simulink model "sensor_diagnosis"  (R2018b)
settings: Solver=FixedStepAuto  StartTime=0.0  StopTime=2000  FixedStep=0.02  RelTol=1e-3
values from neighbouring files (symbols this model uses):
  R = 0.003*eye(size(C,1))    [Com_of_kalman_gain.m]    (also in Copy_of_kalman_gain.m = diag(y_noise.^2); MM_HKF.m = diag(y_svar.^2); MM_based.m = diag(y_svar.^2); act_fault_of_kalman_gain.m = 0.02^2*eye(size(C,1)))
undefined symbols (not defined in the file or in its folder): piece
libraries: sharedschedule x121, dspsigattribs x22, commchan3 x1, dsparch4 x1, simulink x1
(part 2 of 2)

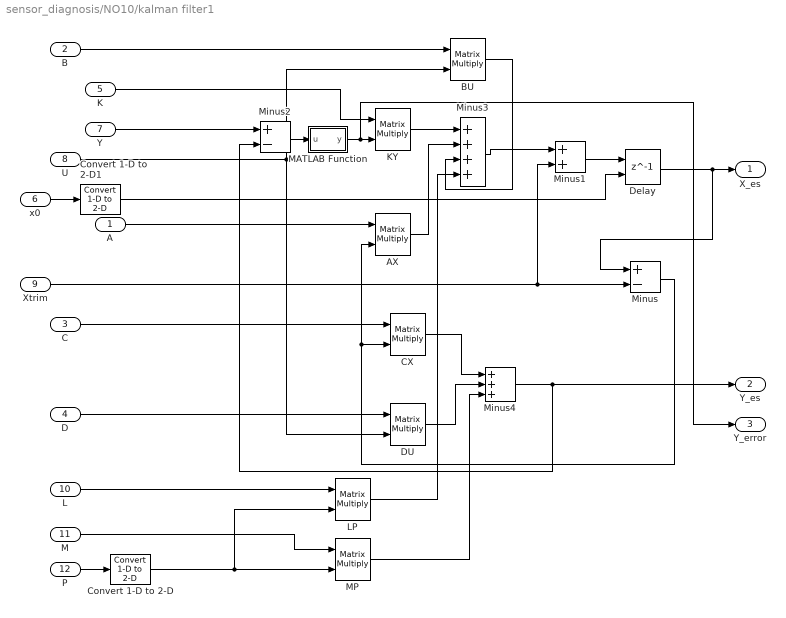
== system sensor_diagnosis/NO10/kalman filter1 ==
  A : Inport
  B : Inport  Port=2
  C : Inport  Port=3
  D : Inport  Port=4
  K : Inport  Port=5
  x0 : Inport  Port=6
  Y : Inport  Port=7
  U : Inport  Port=8
  Xtrim : Inport  Port=9
  L : Inport  Port=10
  M : Inport  Port=11
  P : Inport  Port=12
  "\tCX" : Product  Multiplication=Matrix(*)
  AX : Product  Multiplication=Matrix(*)
  BU : Product  Multiplication=Matrix(*)
  Convert 1-D to 2-D : dspsigattribs/Convert 1-D to 2-D  M=10  N=1  frameBasedOut=off
      settings: SourceProductName=DSP System Toolbox  SourceProductBaseCode=DS
  Convert 1-D to 2-D1 : dspsigattribs/Convert 1-D to 2-D  M=2  N=1  frameBasedOut=off
      settings: SourceProductName=DSP System Toolbox  SourceProductBaseCode=DS
  DU : Product  Multiplication=Matrix(*)
  Delay : Delay  DelayLength=1  InitialConditionSource=Input port
      settings: InputPortMap=u0,p4
  KY : Product  Multiplication=Matrix(*)
  LP : Product  Multiplication=Matrix(*)
  MATLAB Function : MATLAB Function  TreatAsAtomicUnit=on
  MP : Product  Multiplication=Matrix(*)
  Minus : Sum  Inputs=+-
  Minus1 : Sum
  Minus2 : Sum  Inputs=+-
  Minus3 : Sum  Inputs=++++
  Minus4 : Sum  Inputs=+++
  X_es : Outport
  Y_es : Outport  Port=2
  Y_error : Outport  Port=3
  wires:
  Minus1/1 -> Delay/1
  Minus3/1 -> Minus1/1
  AX/1 -> Minus3/2
  Minus/1 -> "\tCX"/2, AX/2
  Delay/1 -> X_es/1, Minus/1
  Xtrim/1 -> Minus/2, Minus1/2
  K/1 -> KY/1
  D/1 -> DU/1
  C/1 -> "\tCX"/1
  B/1 -> BU/1
  A/1 -> AX/1
  BU/1 -> Minus3/3
  "\tCX"/1 -> Minus4/1
  DU/1 -> Minus4/2
  Y/1 -> Minus2/1
  U/1 -> DU/2, BU/2
  KY/1 -> Minus3/1
  Minus4/1 -> Y_es/1, Minus2/2
  L/1 -> LP/1
  M/1 -> MP/1
  LP/1 -> Minus3/4
  MP/1 -> Minus4/3
  P/1 -> Convert 1-D to 2-D/1
  Convert 1-D to 2-D/1 -> LP/2, MP/2
  x0/1 -> Convert 1-D to 2-D1/1
  Convert 1-D to 2-D1/1 -> Delay/2
  Minus2/1 -> MATLAB Function/1(u)
  MATLAB Function/1(y) -> Y_error/1, KY/2

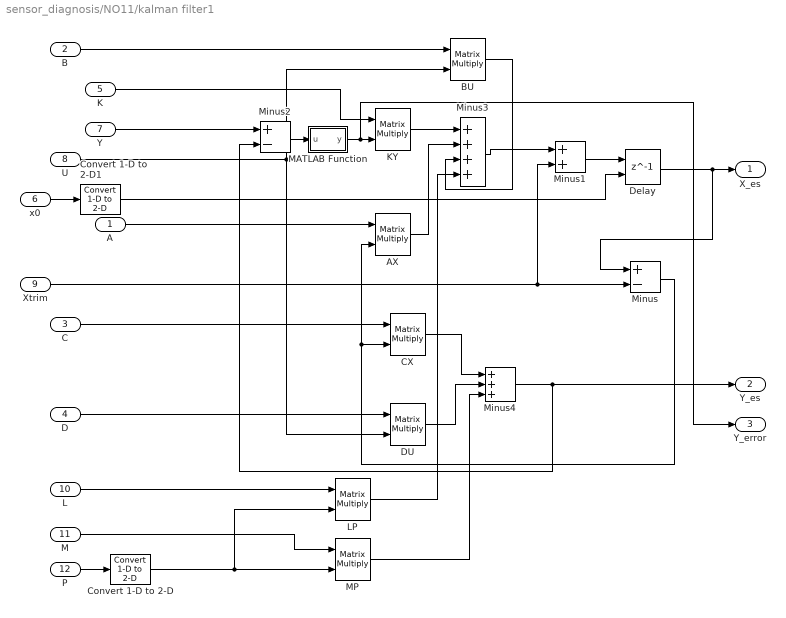
== system sensor_diagnosis/NO11/kalman filter1 ==
  A : Inport
  B : Inport  Port=2
  C : Inport  Port=3
  D : Inport  Port=4
  K : Inport  Port=5
  x0 : Inport  Port=6
  Y : Inport  Port=7
  U : Inport  Port=8
  Xtrim : Inport  Port=9
  L : Inport  Port=10
  M : Inport  Port=11
  P : Inport  Port=12
  "\tCX" : Product  Multiplication=Matrix(*)
  AX : Product  Multiplication=Matrix(*)
  BU : Product  Multiplication=Matrix(*)
  Convert 1-D to 2-D : dspsigattribs/Convert 1-D to 2-D  M=10  N=1  frameBasedOut=off
      settings: SourceProductName=DSP System Toolbox  SourceProductBaseCode=DS
  Convert 1-D to 2-D1 : dspsigattribs/Convert 1-D to 2-D  M=2  N=1  frameBasedOut=off
      settings: SourceProductName=DSP System Toolbox  SourceProductBaseCode=DS
  DU : Product  Multiplication=Matrix(*)
  Delay : Delay  DelayLength=1  InitialConditionSource=Input port
      settings: InputPortMap=u0,p4
  KY : Product  Multiplication=Matrix(*)
  LP : Product  Multiplication=Matrix(*)
  MATLAB Function : MATLAB Function  TreatAsAtomicUnit=on
  MP : Product  Multiplication=Matrix(*)
  Minus : Sum  Inputs=+-
  Minus1 : Sum
  Minus2 : Sum  Inputs=+-
  Minus3 : Sum  Inputs=++++
  Minus4 : Sum  Inputs=+++
  X_es : Outport
  Y_es : Outport  Port=2
  Y_error : Outport  Port=3
  wires:
  MATLAB Function/1(y) -> KY/2, Y_error/1
  Minus2/1 -> MATLAB Function/1(u)
  Convert 1-D to 2-D1/1 -> Delay/2
  x0/1 -> Convert 1-D to 2-D1/1
  Convert 1-D to 2-D/1 -> MP/2, LP/2
  P/1 -> Convert 1-D to 2-D/1
  MP/1 -> Minus4/3
  LP/1 -> Minus3/4
  M/1 -> MP/1
  L/1 -> LP/1
  Minus4/1 -> Minus2/2, Y_es/1
  KY/1 -> Minus3/1
  U/1 -> BU/2, DU/2
  Y/1 -> Minus2/1
  DU/1 -> Minus4/2
  "\tCX"/1 -> Minus4/1
  BU/1 -> Minus3/3
  A/1 -> AX/1
  B/1 -> BU/1
  C/1 -> "\tCX"/1
  D/1 -> DU/1
  K/1 -> KY/1
  Xtrim/1 -> Minus1/2, Minus/2
  Delay/1 -> Minus/1, X_es/1
  Minus/1 -> AX/2, "\tCX"/2
  AX/1 -> Minus3/2
  Minus3/1 -> Minus1/1
  Minus1/1 -> Delay/1

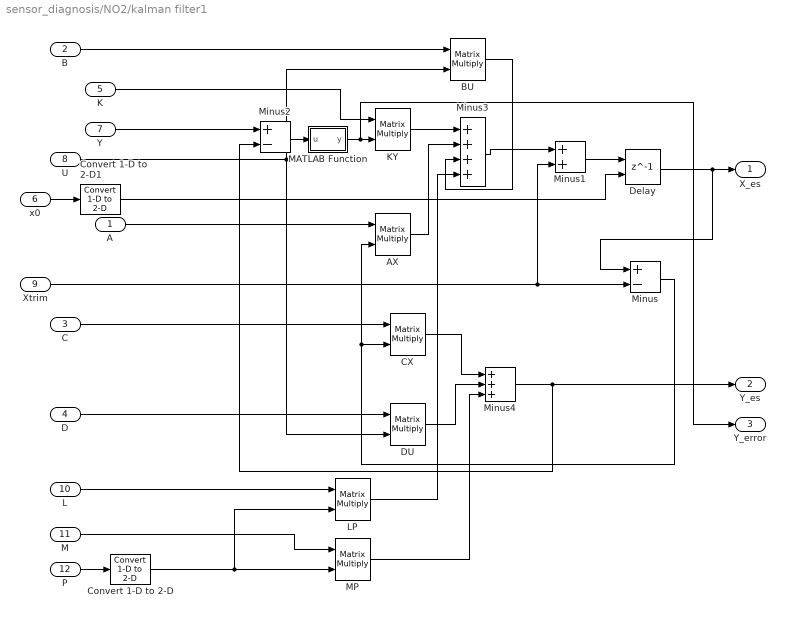
== system sensor_diagnosis/NO2/kalman filter1 ==
  A : Inport
  B : Inport  Port=2
  C : Inport  Port=3
  D : Inport  Port=4
  K : Inport  Port=5
  x0 : Inport  Port=6
  Y : Inport  Port=7
  U : Inport  Port=8
  Xtrim : Inport  Port=9
  L : Inport  Port=10
  M : Inport  Port=11
  P : Inport  Port=12
  "\tCX" : Product  Multiplication=Matrix(*)
  AX : Product  Multiplication=Matrix(*)
  BU : Product  Multiplication=Matrix(*)
  Convert 1-D to 2-D : dspsigattribs/Convert 1-D to 2-D  M=10  N=1  frameBasedOut=off
      settings: SourceProductName=DSP System Toolbox  SourceProductBaseCode=DS
  Convert 1-D to 2-D1 : dspsigattribs/Convert 1-D to 2-D  M=2  N=1  frameBasedOut=off
      settings: SourceProductName=DSP System Toolbox  SourceProductBaseCode=DS
  DU : Product  Multiplication=Matrix(*)
  Delay : Delay  DelayLength=1  InitialConditionSource=Input port
      settings: InputPortMap=u0,p4
  KY : Product  Multiplication=Matrix(*)
  LP : Product  Multiplication=Matrix(*)
  MATLAB Function : MATLAB Function  TreatAsAtomicUnit=on
  MP : Product  Multiplication=Matrix(*)
  Minus : Sum  Inputs=+-
  Minus1 : Sum
  Minus2 : Sum  Inputs=+-
  Minus3 : Sum  Inputs=++++
  Minus4 : Sum  Inputs=+++
  X_es : Outport
  Y_es : Outport  Port=2
  Y_error : Outport  Port=3
  wires:
  Minus1/1 -> Delay/1
  Minus3/1 -> Minus1/1
  AX/1 -> Minus3/2
  Minus/1 -> "\tCX"/2, AX/2
  Delay/1 -> X_es/1, Minus/1
  Xtrim/1 -> Minus/2, Minus1/2
  K/1 -> KY/1
  D/1 -> DU/1
  C/1 -> "\tCX"/1
  B/1 -> BU/1
  A/1 -> AX/1
  BU/1 -> Minus3/3
  "\tCX"/1 -> Minus4/1
  DU/1 -> Minus4/2
  Y/1 -> Minus2/1
  U/1 -> DU/2, BU/2
  KY/1 -> Minus3/1
  Minus4/1 -> Y_es/1, Minus2/2
  L/1 -> LP/1
  M/1 -> MP/1
  LP/1 -> Minus3/4
  MP/1 -> Minus4/3
  P/1 -> Convert 1-D to 2-D/1
  Convert 1-D to 2-D/1 -> LP/2, MP/2
  x0/1 -> Convert 1-D to 2-D1/1
  Convert 1-D to 2-D1/1 -> Delay/2
  Minus2/1 -> MATLAB Function/1(u)
  MATLAB Function/1(y) -> Y_error/1, KY/2

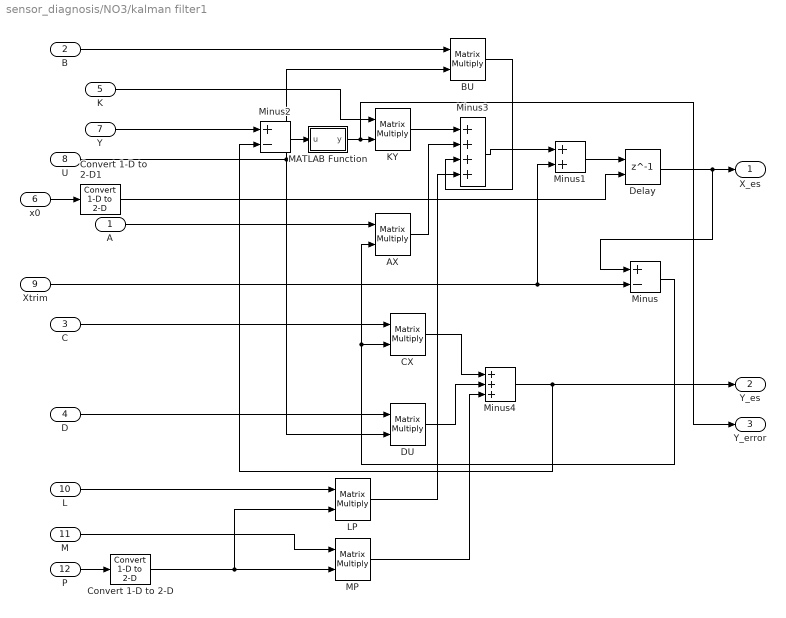
== system sensor_diagnosis/NO3/kalman filter1 ==
  A : Inport
  B : Inport  Port=2
  C : Inport  Port=3
  D : Inport  Port=4
  K : Inport  Port=5
  x0 : Inport  Port=6
  Y : Inport  Port=7
  U : Inport  Port=8
  Xtrim : Inport  Port=9
  L : Inport  Port=10
  M : Inport  Port=11
  P : Inport  Port=12
  "\tCX" : Product  Multiplication=Matrix(*)
  AX : Product  Multiplication=Matrix(*)
  BU : Product  Multiplication=Matrix(*)
  Convert 1-D to 2-D : dspsigattribs/Convert 1-D to 2-D  M=10  N=1  frameBasedOut=off
      settings: SourceProductName=DSP System Toolbox  SourceProductBaseCode=DS
  Convert 1-D to 2-D1 : dspsigattribs/Convert 1-D to 2-D  M=2  N=1  frameBasedOut=off
      settings: SourceProductName=DSP System Toolbox  SourceProductBaseCode=DS
  DU : Product  Multiplication=Matrix(*)
  Delay : Delay  DelayLength=1  InitialConditionSource=Input port
      settings: InputPortMap=u0,p4
  KY : Product  Multiplication=Matrix(*)
  LP : Product  Multiplication=Matrix(*)
  MATLAB Function : MATLAB Function  TreatAsAtomicUnit=on
  MP : Product  Multiplication=Matrix(*)
  Minus : Sum  Inputs=+-
  Minus1 : Sum
  Minus2 : Sum  Inputs=+-
  Minus3 : Sum  Inputs=++++
  Minus4 : Sum  Inputs=+++
  X_es : Outport
  Y_es : Outport  Port=2
  Y_error : Outport  Port=3
  wires:
  Minus1/1 -> Delay/1
  Minus3/1 -> Minus1/1
  AX/1 -> Minus3/2
  Minus/1 -> "\tCX"/2, AX/2
  Delay/1 -> X_es/1, Minus/1
  Xtrim/1 -> Minus/2, Minus1/2
  K/1 -> KY/1
  D/1 -> DU/1
  C/1 -> "\tCX"/1
  B/1 -> BU/1
  A/1 -> AX/1
  BU/1 -> Minus3/3
  "\tCX"/1 -> Minus4/1
  DU/1 -> Minus4/2
  Y/1 -> Minus2/1
  U/1 -> DU/2, BU/2
  KY/1 -> Minus3/1
  Minus4/1 -> Y_es/1, Minus2/2
  L/1 -> LP/1
  M/1 -> MP/1
  LP/1 -> Minus3/4
  MP/1 -> Minus4/3
  P/1 -> Convert 1-D to 2-D/1
  Convert 1-D to 2-D/1 -> LP/2, MP/2
  x0/1 -> Convert 1-D to 2-D1/1
  Convert 1-D to 2-D1/1 -> Delay/2
  Minus2/1 -> MATLAB Function/1(u)
  MATLAB Function/1(y) -> Y_error/1, KY/2

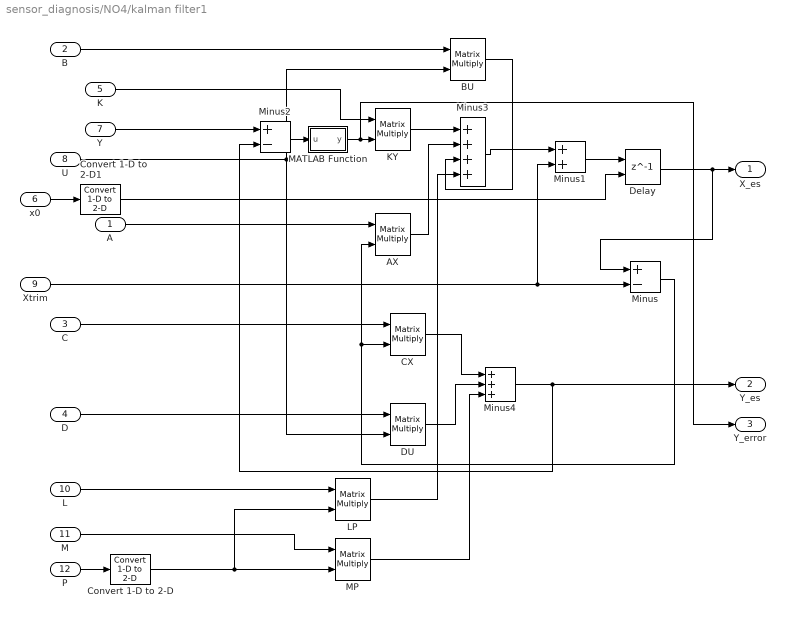
== system sensor_diagnosis/NO4/kalman filter1 ==
  A : Inport
  B : Inport  Port=2
  C : Inport  Port=3
  D : Inport  Port=4
  K : Inport  Port=5
  x0 : Inport  Port=6
  Y : Inport  Port=7
  U : Inport  Port=8
  Xtrim : Inport  Port=9
  L : Inport  Port=10
  M : Inport  Port=11
  P : Inport  Port=12
  "\tCX" : Product  Multiplication=Matrix(*)
  AX : Product  Multiplication=Matrix(*)
  BU : Product  Multiplication=Matrix(*)
  Convert 1-D to 2-D : dspsigattribs/Convert 1-D to 2-D  M=10  N=1  frameBasedOut=off
      settings: SourceProductName=DSP System Toolbox  SourceProductBaseCode=DS
  Convert 1-D to 2-D1 : dspsigattribs/Convert 1-D to 2-D  M=2  N=1  frameBasedOut=off
      settings: SourceProductName=DSP System Toolbox  SourceProductBaseCode=DS
  DU : Product  Multiplication=Matrix(*)
  Delay : Delay  DelayLength=1  InitialConditionSource=Input port
      settings: InputPortMap=u0,p4
  KY : Product  Multiplication=Matrix(*)
  LP : Product  Multiplication=Matrix(*)
  MATLAB Function : MATLAB Function  TreatAsAtomicUnit=on
  MP : Product  Multiplication=Matrix(*)
  Minus : Sum  Inputs=+-
  Minus1 : Sum
  Minus2 : Sum  Inputs=+-
  Minus3 : Sum  Inputs=++++
  Minus4 : Sum  Inputs=+++
  X_es : Outport
  Y_es : Outport  Port=2
  Y_error : Outport  Port=3
  wires:
  Minus1/1 -> Delay/1
  Minus3/1 -> Minus1/1
  AX/1 -> Minus3/2
  Minus/1 -> "\tCX"/2, AX/2
  Delay/1 -> X_es/1, Minus/1
  Xtrim/1 -> Minus/2, Minus1/2
  K/1 -> KY/1
  D/1 -> DU/1
  C/1 -> "\tCX"/1
  B/1 -> BU/1
  A/1 -> AX/1
  BU/1 -> Minus3/3
  "\tCX"/1 -> Minus4/1
  DU/1 -> Minus4/2
  Y/1 -> Minus2/1
  U/1 -> DU/2, BU/2
  KY/1 -> Minus3/1
  Minus4/1 -> Y_es/1, Minus2/2
  L/1 -> LP/1
  M/1 -> MP/1
  LP/1 -> Minus3/4
  MP/1 -> Minus4/3
  P/1 -> Convert 1-D to 2-D/1
  Convert 1-D to 2-D/1 -> LP/2, MP/2
  x0/1 -> Convert 1-D to 2-D1/1
  Convert 1-D to 2-D1/1 -> Delay/2
  Minus2/1 -> MATLAB Function/1(u)
  MATLAB Function/1(y) -> Y_error/1, KY/2

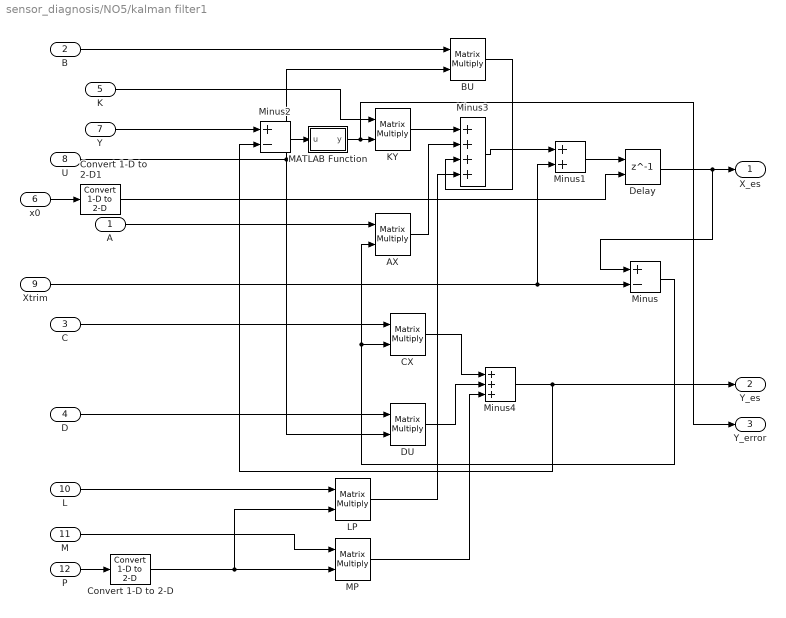
== system sensor_diagnosis/NO5/kalman filter1 ==
  A : Inport
  B : Inport  Port=2
  C : Inport  Port=3
  D : Inport  Port=4
  K : Inport  Port=5
  x0 : Inport  Port=6
  Y : Inport  Port=7
  U : Inport  Port=8
  Xtrim : Inport  Port=9
  L : Inport  Port=10
  M : Inport  Port=11
  P : Inport  Port=12
  "\tCX" : Product  Multiplication=Matrix(*)
  AX : Product  Multiplication=Matrix(*)
  BU : Product  Multiplication=Matrix(*)
  Convert 1-D to 2-D : dspsigattribs/Convert 1-D to 2-D  M=10  N=1  frameBasedOut=off
      settings: SourceProductName=DSP System Toolbox  SourceProductBaseCode=DS
  Convert 1-D to 2-D1 : dspsigattribs/Convert 1-D to 2-D  M=2  N=1  frameBasedOut=off
      settings: SourceProductName=DSP System Toolbox  SourceProductBaseCode=DS
  DU : Product  Multiplication=Matrix(*)
  Delay : Delay  DelayLength=1  InitialConditionSource=Input port
      settings: InputPortMap=u0,p4
  KY : Product  Multiplication=Matrix(*)
  LP : Product  Multiplication=Matrix(*)
  MATLAB Function : MATLAB Function  TreatAsAtomicUnit=on
  MP : Product  Multiplication=Matrix(*)
  Minus : Sum  Inputs=+-
  Minus1 : Sum
  Minus2 : Sum  Inputs=+-
  Minus3 : Sum  Inputs=++++
  Minus4 : Sum  Inputs=+++
  X_es : Outport
  Y_es : Outport  Port=2
  Y_error : Outport  Port=3
  wires:
  Minus1/1 -> Delay/1
  Minus3/1 -> Minus1/1
  AX/1 -> Minus3/2
  Minus/1 -> "\tCX"/2, AX/2
  Delay/1 -> X_es/1, Minus/1
  Xtrim/1 -> Minus/2, Minus1/2
  K/1 -> KY/1
  D/1 -> DU/1
  C/1 -> "\tCX"/1
  B/1 -> BU/1
  A/1 -> AX/1
  BU/1 -> Minus3/3
  "\tCX"/1 -> Minus4/1
  DU/1 -> Minus4/2
  Y/1 -> Minus2/1
  U/1 -> DU/2, BU/2
  KY/1 -> Minus3/1
  Minus4/1 -> Y_es/1, Minus2/2
  L/1 -> LP/1
  M/1 -> MP/1
  LP/1 -> Minus3/4
  MP/1 -> Minus4/3
  P/1 -> Convert 1-D to 2-D/1
  Convert 1-D to 2-D/1 -> LP/2, MP/2
  x0/1 -> Convert 1-D to 2-D1/1
  Convert 1-D to 2-D1/1 -> Delay/2
  Minus2/1 -> MATLAB Function/1(u)
  MATLAB Function/1(y) -> Y_error/1, KY/2

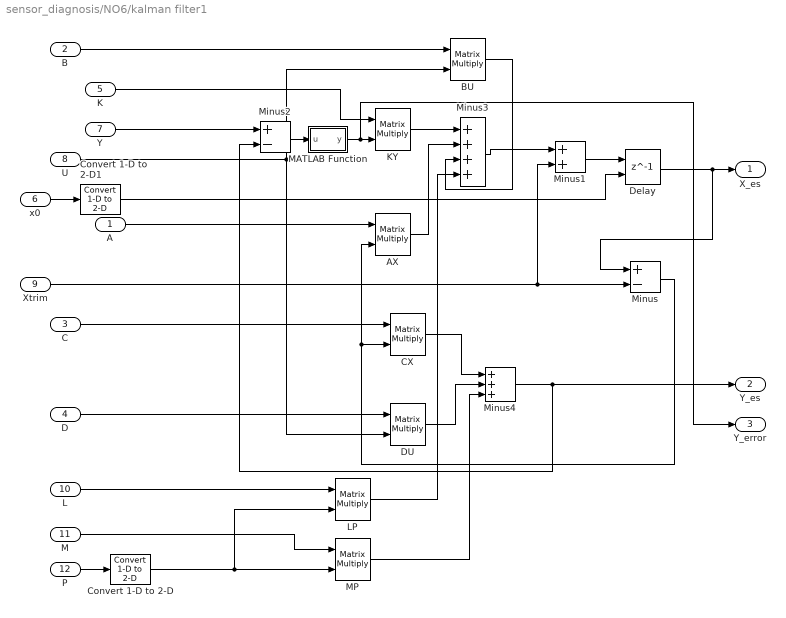
== system sensor_diagnosis/NO6/kalman filter1 ==
  A : Inport
  B : Inport  Port=2
  C : Inport  Port=3
  D : Inport  Port=4
  K : Inport  Port=5
  x0 : Inport  Port=6
  Y : Inport  Port=7
  U : Inport  Port=8
  Xtrim : Inport  Port=9
  L : Inport  Port=10
  M : Inport  Port=11
  P : Inport  Port=12
  "\tCX" : Product  Multiplication=Matrix(*)
  AX : Product  Multiplication=Matrix(*)
  BU : Product  Multiplication=Matrix(*)
  Convert 1-D to 2-D : dspsigattribs/Convert 1-D to 2-D  M=10  N=1  frameBasedOut=off
      settings: SourceProductName=DSP System Toolbox  SourceProductBaseCode=DS
  Convert 1-D to 2-D1 : dspsigattribs/Convert 1-D to 2-D  M=2  N=1  frameBasedOut=off
      settings: SourceProductName=DSP System Toolbox  SourceProductBaseCode=DS
  DU : Product  Multiplication=Matrix(*)
  Delay : Delay  DelayLength=1  InitialConditionSource=Input port
      settings: InputPortMap=u0,p4
  KY : Product  Multiplication=Matrix(*)
  LP : Product  Multiplication=Matrix(*)
  MATLAB Function : MATLAB Function  TreatAsAtomicUnit=on
  MP : Product  Multiplication=Matrix(*)
  Minus : Sum  Inputs=+-
  Minus1 : Sum
  Minus2 : Sum  Inputs=+-
  Minus3 : Sum  Inputs=++++
  Minus4 : Sum  Inputs=+++
  X_es : Outport
  Y_es : Outport  Port=2
  Y_error : Outport  Port=3
  wires:
  Minus1/1 -> Delay/1
  Minus3/1 -> Minus1/1
  AX/1 -> Minus3/2
  Minus/1 -> "\tCX"/2, AX/2
  Delay/1 -> X_es/1, Minus/1
  Xtrim/1 -> Minus/2, Minus1/2
  K/1 -> KY/1
  D/1 -> DU/1
  C/1 -> "\tCX"/1
  B/1 -> BU/1
  A/1 -> AX/1
  BU/1 -> Minus3/3
  "\tCX"/1 -> Minus4/1
  DU/1 -> Minus4/2
  Y/1 -> Minus2/1
  U/1 -> DU/2, BU/2
  KY/1 -> Minus3/1
  Minus4/1 -> Y_es/1, Minus2/2
  L/1 -> LP/1
  M/1 -> MP/1
  LP/1 -> Minus3/4
  MP/1 -> Minus4/3
  P/1 -> Convert 1-D to 2-D/1
  Convert 1-D to 2-D/1 -> LP/2, MP/2
  x0/1 -> Convert 1-D to 2-D1/1
  Convert 1-D to 2-D1/1 -> Delay/2
  Minus2/1 -> MATLAB Function/1(u)
  MATLAB Function/1(y) -> Y_error/1, KY/2

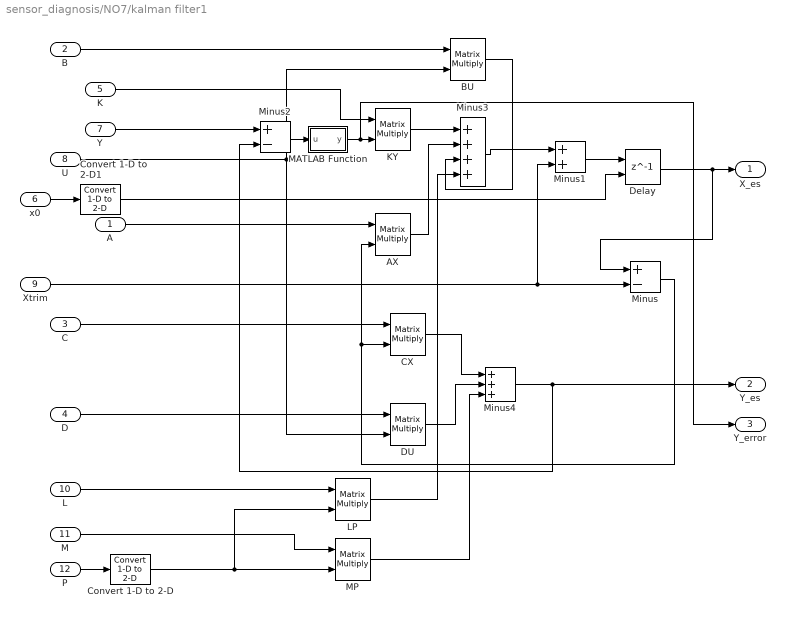
== system sensor_diagnosis/NO7/kalman filter1 ==
  A : Inport
  B : Inport  Port=2
  C : Inport  Port=3
  D : Inport  Port=4
  K : Inport  Port=5
  x0 : Inport  Port=6
  Y : Inport  Port=7
  U : Inport  Port=8
  Xtrim : Inport  Port=9
  L : Inport  Port=10
  M : Inport  Port=11
  P : Inport  Port=12
  "\tCX" : Product  Multiplication=Matrix(*)
  AX : Product  Multiplication=Matrix(*)
  BU : Product  Multiplication=Matrix(*)
  Convert 1-D to 2-D : dspsigattribs/Convert 1-D to 2-D  M=10  N=1  frameBasedOut=off
      settings: SourceProductName=DSP System Toolbox  SourceProductBaseCode=DS
  Convert 1-D to 2-D1 : dspsigattribs/Convert 1-D to 2-D  M=2  N=1  frameBasedOut=off
      settings: SourceProductName=DSP System Toolbox  SourceProductBaseCode=DS
  DU : Product  Multiplication=Matrix(*)
  Delay : Delay  DelayLength=1  InitialConditionSource=Input port
      settings: InputPortMap=u0,p4
  KY : Product  Multiplication=Matrix(*)
  LP : Product  Multiplication=Matrix(*)
  MATLAB Function : MATLAB Function  TreatAsAtomicUnit=on
  MP : Product  Multiplication=Matrix(*)
  Minus : Sum  Inputs=+-
  Minus1 : Sum
  Minus2 : Sum  Inputs=+-
  Minus3 : Sum  Inputs=++++
  Minus4 : Sum  Inputs=+++
  X_es : Outport
  Y_es : Outport  Port=2
  Y_error : Outport  Port=3
  wires:
  Minus1/1 -> Delay/1
  Minus3/1 -> Minus1/1
  AX/1 -> Minus3/2
  Minus/1 -> "\tCX"/2, AX/2
  Delay/1 -> X_es/1, Minus/1
  Xtrim/1 -> Minus/2, Minus1/2
  K/1 -> KY/1
  D/1 -> DU/1
  C/1 -> "\tCX"/1
  B/1 -> BU/1
  A/1 -> AX/1
  BU/1 -> Minus3/3
  "\tCX"/1 -> Minus4/1
  DU/1 -> Minus4/2
  Y/1 -> Minus2/1
  U/1 -> DU/2, BU/2
  KY/1 -> Minus3/1
  Minus4/1 -> Y_es/1, Minus2/2
  L/1 -> LP/1
  M/1 -> MP/1
  LP/1 -> Minus3/4
  MP/1 -> Minus4/3
  P/1 -> Convert 1-D to 2-D/1
  Convert 1-D to 2-D/1 -> LP/2, MP/2
  x0/1 -> Convert 1-D to 2-D1/1
  Convert 1-D to 2-D1/1 -> Delay/2
  Minus2/1 -> MATLAB Function/1(u)
  MATLAB Function/1(y) -> Y_error/1, KY/2

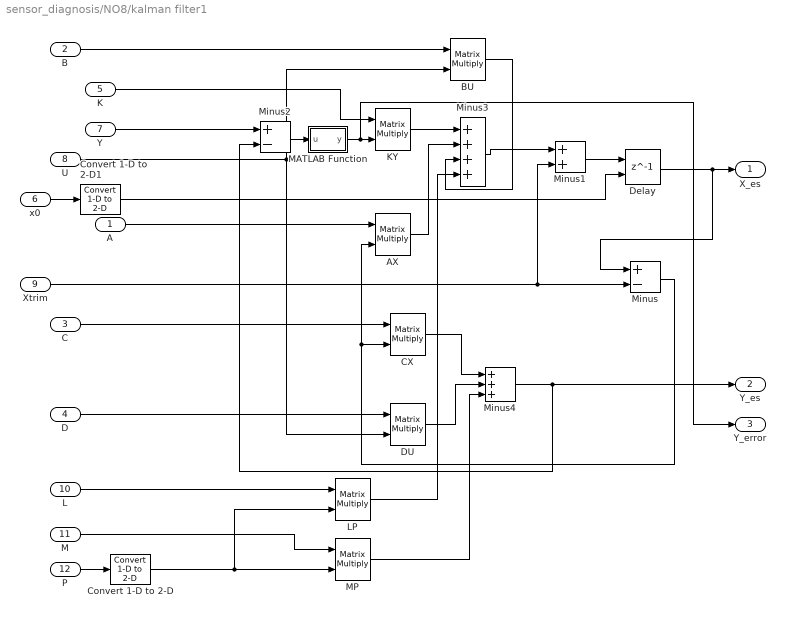
== system sensor_diagnosis/NO8/kalman filter1 ==
  A : Inport
  B : Inport  Port=2
  C : Inport  Port=3
  D : Inport  Port=4
  K : Inport  Port=5
  x0 : Inport  Port=6
  Y : Inport  Port=7
  U : Inport  Port=8
  Xtrim : Inport  Port=9
  L : Inport  Port=10
  M : Inport  Port=11
  P : Inport  Port=12
  "\tCX" : Product  Multiplication=Matrix(*)
  AX : Product  Multiplication=Matrix(*)
  BU : Product  Multiplication=Matrix(*)
  Convert 1-D to 2-D : dspsigattribs/Convert 1-D to 2-D  M=10  N=1  frameBasedOut=off
      settings: SourceProductName=DSP System Toolbox  SourceProductBaseCode=DS
  Convert 1-D to 2-D1 : dspsigattribs/Convert 1-D to 2-D  M=2  N=1  frameBasedOut=off
      settings: SourceProductName=DSP System Toolbox  SourceProductBaseCode=DS
  DU : Product  Multiplication=Matrix(*)
  Delay : Delay  DelayLength=1  InitialConditionSource=Input port
      settings: InputPortMap=u0,p4
  KY : Product  Multiplication=Matrix(*)
  LP : Product  Multiplication=Matrix(*)
  MATLAB Function : MATLAB Function  TreatAsAtomicUnit=on
  MP : Product  Multiplication=Matrix(*)
  Minus : Sum  Inputs=+-
  Minus1 : Sum
  Minus2 : Sum  Inputs=+-
  Minus3 : Sum  Inputs=++++
  Minus4 : Sum  Inputs=+++
  X_es : Outport
  Y_es : Outport  Port=2
  Y_error : Outport  Port=3
  wires:
  Minus1/1 -> Delay/1
  Minus3/1 -> Minus1/1
  AX/1 -> Minus3/2
  Minus/1 -> "\tCX"/2, AX/2
  Delay/1 -> X_es/1, Minus/1
  Xtrim/1 -> Minus/2, Minus1/2
  K/1 -> KY/1
  D/1 -> DU/1
  C/1 -> "\tCX"/1
  B/1 -> BU/1
  A/1 -> AX/1
  BU/1 -> Minus3/3
  "\tCX"/1 -> Minus4/1
  DU/1 -> Minus4/2
  Y/1 -> Minus2/1
  U/1 -> DU/2, BU/2
  KY/1 -> Minus3/1
  Minus4/1 -> Y_es/1, Minus2/2
  L/1 -> LP/1
  M/1 -> MP/1
  LP/1 -> Minus3/4
  MP/1 -> Minus4/3
  P/1 -> Convert 1-D to 2-D/1
  Convert 1-D to 2-D/1 -> LP/2, MP/2
  x0/1 -> Convert 1-D to 2-D1/1
  Convert 1-D to 2-D1/1 -> Delay/2
  Minus2/1 -> MATLAB Function/1(u)
  MATLAB Function/1(y) -> Y_error/1, KY/2

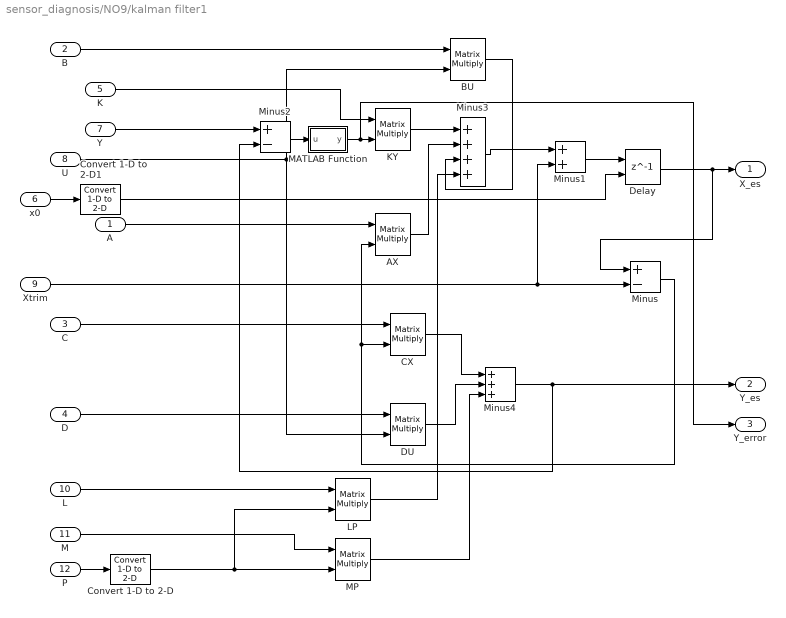
== system sensor_diagnosis/NO9/kalman filter1 ==
  A : Inport
  B : Inport  Port=2
  C : Inport  Port=3
  D : Inport  Port=4
  K : Inport  Port=5
  x0 : Inport  Port=6
  Y : Inport  Port=7
  U : Inport  Port=8
  Xtrim : Inport  Port=9
  L : Inport  Port=10
  M : Inport  Port=11
  P : Inport  Port=12
  "\tCX" : Product  Multiplication=Matrix(*)
  AX : Product  Multiplication=Matrix(*)
  BU : Product  Multiplication=Matrix(*)
  Convert 1-D to 2-D : dspsigattribs/Convert 1-D to 2-D  M=10  N=1  frameBasedOut=off
      settings: SourceProductName=DSP System Toolbox  SourceProductBaseCode=DS
  Convert 1-D to 2-D1 : dspsigattribs/Convert 1-D to 2-D  M=2  N=1  frameBasedOut=off
      settings: SourceProductName=DSP System Toolbox  SourceProductBaseCode=DS
  DU : Product  Multiplication=Matrix(*)
  Delay : Delay  DelayLength=1  InitialConditionSource=Input port
      settings: InputPortMap=u0,p4
  KY : Product  Multiplication=Matrix(*)
  LP : Product  Multiplication=Matrix(*)
  MATLAB Function : MATLAB Function  TreatAsAtomicUnit=on
  MP : Product  Multiplication=Matrix(*)
  Minus : Sum  Inputs=+-
  Minus1 : Sum
  Minus2 : Sum  Inputs=+-
  Minus3 : Sum  Inputs=++++
  Minus4 : Sum  Inputs=+++
  X_es : Outport
  Y_es : Outport  Port=2
  Y_error : Outport  Port=3
  wires:
  Minus1/1 -> Delay/1
  Minus3/1 -> Minus1/1
  AX/1 -> Minus3/2
  Minus/1 -> "\tCX"/2, AX/2
  Delay/1 -> X_es/1, Minus/1
  Xtrim/1 -> Minus/2, Minus1/2
  K/1 -> KY/1
  D/1 -> DU/1
  C/1 -> "\tCX"/1
  B/1 -> BU/1
  A/1 -> AX/1
  BU/1 -> Minus3/3
  "\tCX"/1 -> Minus4/1
  DU/1 -> Minus4/2
  Y/1 -> Minus2/1
  U/1 -> DU/2, BU/2
  KY/1 -> Minus3/1
  Minus4/1 -> Y_es/1, Minus2/2
  L/1 -> LP/1
  M/1 -> MP/1
  LP/1 -> Minus3/4
  MP/1 -> Minus4/3
  P/1 -> Convert 1-D to 2-D/1
  Convert 1-D to 2-D/1 -> LP/2, MP/2
  x0/1 -> Convert 1-D to 2-D1/1
  Convert 1-D to 2-D1/1 -> Delay/2
  Minus2/1 -> MATLAB Function/1(u)
  MATLAB Function/1(y) -> Y_error/1, KY/2

== matlab function sensor_diagnosis/normlization1 ==
  data: N output; row_data input; P output; T_index input; P_index input; HP_index input; U_index input; N_index input; T output; U output; HP output; TP2 output
function [N,P,T,U,HP,TP2] = fcn(row_data,T_index,P_index,HP_index,U_index,N_index)
%%% 数据相似归一化
% if size(mean_design,1) > size(mean_design,2)
%     mean_ = mean_design';
% else
%     mean_ = mean_design;
% end
if size(T_index,1) > size(T_index,2)
    T_index_ = T_index';
else
    T_index_ = T_index;
end
if size(P_index,1) > size(P_index,2)
    P_index_ = P_index';
else
    P_index_ = P_index;
end
if size(HP_index,1) > size(HP_index,2)
    HP_index_ = HP_index';
else
    HP_index_ = HP_index;
end
if size(U_index,1) > size(U_index,2)
    U_index_ = U_index';
else
    U_index_ = U_index;
end
if size(N_index,1) > size(N_index,2)
    N_index_ = N_index';
else
    N_index_ = N_index;
end
if size(row_data,1)>size(row_data,2)
    row = row_data';
else
    row = row_data;
end
T2_index = 12;
P2_index = 13;
T = row(:,T_index_);
P = row(:,P_index_);
HP = row(:,HP_index_)'-1;
U = row(:,U_index_);
N = row(:,N_index_);

TP2 = row(:,[T2_index ,P2_index]);
% sigma_P = mean_(P_index_)./mean_(P2_index);
% sigma_T = mean_(T_index_)./mean_(T2_index);
% sigma_Wf = mean_(U_index_(:,1)).*sqrt(mean_(T2_index))./mean_(P2_index);
% sigma_N = mean_(N_index_)./mean_(T2_index);
% Tn = [(T./row(:,T2_index))./sigma_T]';
% Pn = [(P./row(:,P2_index))./sigma_P]';
% Wfn = (U(:,1).*sqrt(row(:,T2_index))./row(:,P2_index))./sigma_Wf;
% Nn = [N./row(:,T2_index)./sigma_N]';
% Un = [Wfn,U(:,2:end)]';

== matlab function sensor_diagnosis/NO1/kalman filter1/MATLAB Function ==
  data: u input; y output
function y = fcn(u)
u(1) = 0;
y = u;

== matlab function sensor_diagnosis/normlization2 ==
  data: Nn output; Pn output; row_data input; Tn output; T_index input; P_index input; HP_index input; U_index input; N_index input; TP2 input; mean_design input; Wfn output; Un output; HP output
function [Nn,Pn,Tn,Wfn,Un,HP] = fcn(row_data,T_index,P_index,HP_index,U_index,N_index,TP2,mean_design)
%%% 数据相似归一化
if size(mean_design,1) > size(mean_design,2)
    mean_ = mean_design';
else
    mean_ = mean_design;
end
if size(T_index,1) > size(T_index,2)
    T_index_ = T_index';
else
    T_index_ = T_index;
end
if size(P_index,1) > size(P_index,2)
    P_index_ = P_index';
else
    P_index_ = P_index;
end
if size(HP_index,1) > size(HP_index,2)
    HP_index_ = HP_index';
else
    HP_index_ = HP_index;
end
if size(U_index,1) > size(U_index,2)
    U_index_ = U_index';
else
    U_index_ = U_index;
end
if size(N_index,1) > size(N_index,2)
    N_index_ = N_index';
else
    N_index_ = N_index;
end
if size(row_data,1)>size(row_data,2)
    row = row_data';
else
    row = row_data;
end
N_len = length(N_index);
T_len = length(T_index);
P_len = length(P_index);
U_len = length(U_index);
HP_len = length(HP_index);
T2_index = 12;
P2_index = 13;
T = row(:,N_len+P_len+1:N_len+P_len+T_len);
P = row(:,N_len+1:N_len+P_len);
HP = row(:,N_len+P_len+T_len+U_len+1:end)'-1;
U = row(:,N_len+P_len+T_len+1:N_len+P_len+T_len+U_len);
N = row(:,1:N_len);
sigma_P = mean_(P_index_)./mean_(P2_index);
sigma_T = mean_(T_index_)./mean_(T2_index);
sigma_Wf = mean_(U_index_(:,1)).*sqrt(mean_(T2_index))./mean_(P2_index);
sigma_N = mean_(N_index_)./mean_(T2_index);
Tn = [(T./TP2(1))./sigma_T]';
Pn = [(P./TP2(2))./sigma_P]';
Wfn = (U(:,1).*sqrt(TP2(1))./TP2(2))./sigma_Wf;
Nn = [N./TP2(1)./sigma_N]';
Un = [Wfn,U(:,2:end)]';

end

== matlab function sensor_diagnosis/normlization3 ==
  data: N output; row_data input; P output; T_index input; P_index input; HP_index input; U_index input; N_index input; T output; U output; HP output; TP2 output
function [N,P,T,U,HP,TP2] = fcn(row_data,T_index,P_index,HP_index,U_index,N_index)
%%% 数据相似归一化
% if size(mean_design,1) > size(mean_design,2)
%     mean_ = mean_design';
% else
%     mean_ = mean_design;
% end
if size(T_index,1) > size(T_index,2)
    T_index_ = T_index';
else
    T_index_ = T_index;
end
if size(P_index,1) > size(P_index,2)
    P_index_ = P_index';
else
    P_index_ = P_index;
end
if size(HP_index,1) > size(HP_index,2)
    HP_index_ = HP_index';
else
    HP_index_ = HP_index;
end
if size(U_index,1) > size(U_index,2)
    U_index_ = U_index';
else
    U_index_ = U_index;
end
if size(N_index,1) > size(N_index,2)
    N_index_ = N_index';
else
    N_index_ = N_index;
end
if size(row_data,1)>size(row_data,2)
    row = row_data';
else
    row = row_data;
end
T2_index = 12;
P2_index = 13;
T = row(:,T_index_);
P = row(:,P_index_);
HP = row(:,HP_index_)'-1;
U = row(:,U_index_);
N = row(:,N_index_);

TP2 = row(:,[T2_index ,P2_index]);
% sigma_P = mean_(P_index_)./mean_(P2_index);
% sigma_T = mean_(T_index_)./mean_(T2_index);
% sigma_Wf = mean_(U_index_(:,1)).*sqrt(mean_(T2_index))./mean_(P2_index);
% sigma_N = mean_(N_index_)./mean_(T2_index);
% Tn = [(T./row(:,T2_index))./sigma_T]';
% Pn = [(P./row(:,P2_index))./sigma_P]';
% Wfn = (U(:,1).*sqrt(row(:,T2_index))./row(:,P2_index))./sigma_Wf;
% Nn = [N./row(:,T2_index)./sigma_N]';
% Un = [Wfn,U(:,2:end)]';

== matlab function sensor_diagnosis/NO2/kalman filter1/MATLAB Function ==
  data: u input; y output
function y = fcn(u)
u(2) = 0;
y = u;

== matlab function sensor_diagnosis/NO3/kalman filter1/MATLAB Function ==
  data: u input; y output
function y = fcn(u)
u(3) = 0;
y = u;

== matlab function sensor_diagnosis/NO4/kalman filter1/MATLAB Function ==
  data: u input; y output
function y = fcn(u)
u(4) = 0;
y = u;

== matlab function sensor_diagnosis/NO5/kalman filter1/MATLAB Function ==
  data: u input; y output
function y = fcn(u)
u(5) = 0;
y = u;

== matlab function sensor_diagnosis/NO6/kalman filter1/MATLAB Function ==
  data: u input; y output
function y = fcn(u)
u(6) = 0;
y = u;

== matlab function sensor_diagnosis/NO7/kalman filter1/MATLAB Function ==
  data: u input; y output
function y = fcn(u)
u(7) = 0;
y = u;

== matlab function sensor_diagnosis/NO8/kalman filter1/MATLAB Function ==
  data: u input; y output
function y = fcn(u)
u(8) = 0;
y = u;

== matlab function sensor_diagnosis/NO9/kalman filter1/MATLAB Function ==
  data: u input; y output
function y = fcn(u)
u(9) = 0;
y = u;

== matlab function sensor_diagnosis/NO10/kalman filter1/MATLAB Function ==
  data: u input; y output
function y = fcn(u)
u(10) = 0;
y = u;

== matlab function sensor_diagnosis/MATLAB Function ==
  data: mag input; y output; no input
function y = fcn(mag,no)
y_ = zeros(1,10);
y_(no) = mag;
y = y_';
end

== matlab function sensor_diagnosis/MATLAB Function1 ==
  data: u input; y output
function y = fcn(u)
%#codegen
u_sum = sum(u);
y = u./u_sum;
if max(y)<=0.99999
    y(1:end-1) = 0;
    y(end) = 1;
end
end

== matlab function sensor_diagnosis/NO11/kalman filter1/MATLAB Function ==
  data: u input; y output
function y = fcn(u)
% u(10) = 0;
y = u;
